simulink model "SLemba_CPG"  (R2024a)
settings: Solver=ode113  StartTime=0.0  StopTime=Sim.time  MaxStep=1e-3  RelTol=1e-5  AbsTol=1e-5
InitFcn:
  | parameters;
  | initBusObjects;
  | loadCPGParam;
undefined symbols (not defined in the file or in its folder): out
settings Model: Creator=heath  LastModifiedBy=Mechatronics
settings SolverCC: ZeroCrossControl=EnableAll
settings DebuggingCC: AlgebraicLoopMsg=none

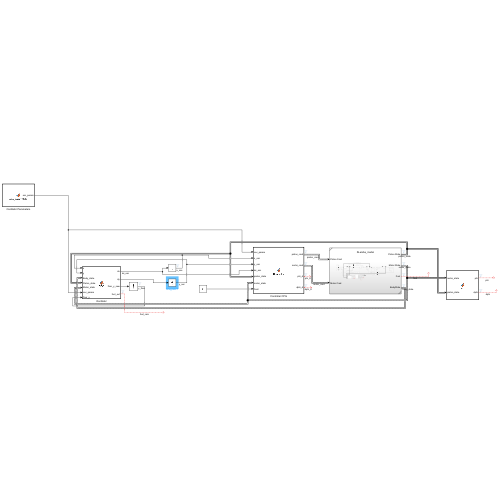
[thumbnail: Simulink's stored preview of the top-level diagram]
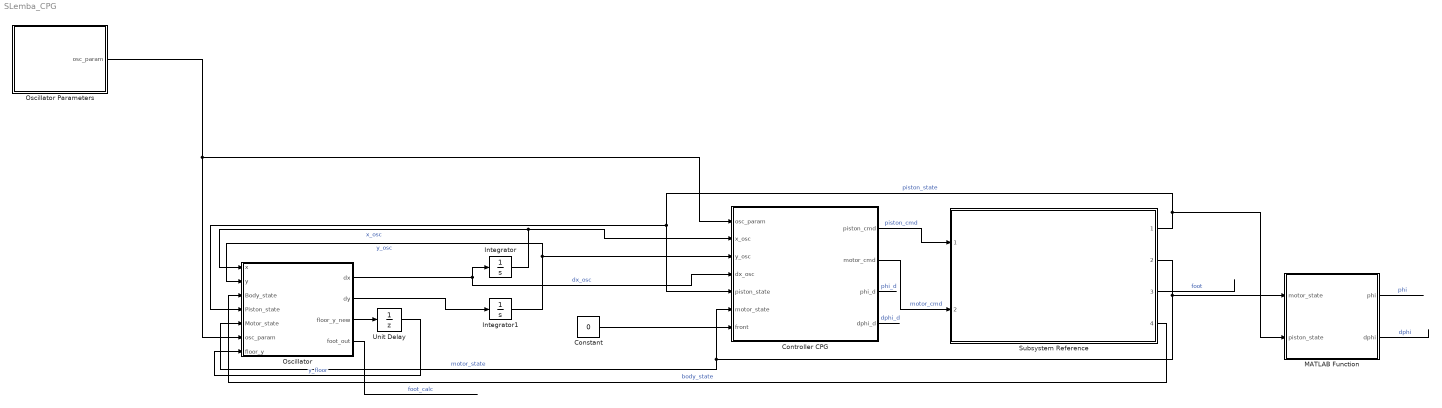
== system SLemba_CPG ==
  Constant : Constant  Value=0
  Controller CPG : MATLAB Function  TreatAsAtomicUnit=on
  Integrator : Integrator  InitialCondition=out.tstInit.CPG(1)
  Integrator1 : Integrator  InitialCondition=out.tstInit.CPG(2)
  MATLAB Function : MATLAB Function  TreatAsAtomicUnit=on
  Oscillator : MATLAB Function  TreatAsAtomicUnit=on
  Oscillator Parameters : MATLAB Function  TreatAsAtomicUnit=on
  Subsystem Reference : Subsystem  ReferencedSubsystem=SLemba_model
  Unit Delay : UnitDelay  SampleTime=-1  HasFrameUpgradeWarning=on
  wires:
  Integrator/1 -> Oscillator/1(x), Controller CPG/2(x_osc)  "x_osc"
  Integrator1/1 -> Oscillator/2(y), Controller CPG/3(y_osc)  "y_osc"
  Subsystem Reference/1 -> MATLAB Function/2(piston_state), Oscillator/4(Piston_state), Controller CPG/5(piston_state)  "piston_state"
  Subsystem Reference/2 -> MATLAB Function/1(motor_state), Oscillator/5(Motor_state), Controller CPG/6(motor_state)  "motor_state"
  Constant/1 -> Controller CPG/7(front)
  Controller CPG/1(piston_cmd) -> Subsystem Reference/1  "piston_cmd"
  Controller CPG/2(motor_cmd) -> Subsystem Reference/2  "motor_cmd"
  Subsystem Reference/4 -> Oscillator/3(Body_state)  "body_state"
  Subsystem Reference/3 -> ?  "foot"
  Controller CPG/3(phi_d) -> ?  "phi_d"
  Controller CPG/4(dphi_d) -> ?  "dphi_d"
  MATLAB Function/1(phi) -> ?  "phi"
  MATLAB Function/2(dphi) -> ?  "dphi"
  Oscillator/1(dx) -> Integrator/1, Controller CPG/4(dx_osc)  "dx_osc"
  Oscillator/2(dy) -> Integrator1/1
  Oscillator/3(floor_y_new) -> Unit Delay/1
  Unit Delay/1 -> Oscillator/7(floor_y)  "y_floor"
  Oscillator/4(foot_out) -> ?  "foot_calc"
  Oscillator Parameters/1(osc_param) -> Oscillator/6(osc_param), Controller CPG/1(osc_param)

== matlab function SLemba_CPG/Controller CPG ==
  data: osc_param input; x_osc input; piston_cmd output Bus: PistonCmd; y_osc input; dx_osc input; piston_state input PistonState; motor_state input MotorState; front input; motor_cmd output Bus: MotorCmd; phi_d output; dphi_d output
function [piston_cmd,motor_cmd,phi_d,dphi_d] = Controller(osc_param, x_osc,y_osc,dx_osc, piston_state,motor_state,front)

kx = osc_param(3);

l = piston_state.p;
dl = piston_state.v;
th = motor_state.q;

if (front)
    direction = -1;
else
    direction = 1;
end

% set command
phi_d = direction*x_osc*kx + pi/2;
dphi_d = direction*dx_osc*kx;
if (y_osc>0) 
    if(x_osc>0)
        ue = 0; ur = 1;
    else
            ue = 1; ur = 1;
    end
else
    ue = 1; ur = 0;
end

kp = 250;
kd = 10;

% % Testing
% % ----------
% ue = 0; ur = 0;
% phi_d = pi/2; dphi_d = 0;
% kp = 250;kd = 5;
% % ---------

piston_cmd.ue = ue;
piston_cmd.ur = ur;

motor_cmd.q = th_calc(phi_d,l);
motor_cmd.w = dth_calc(phi_calc(th,l),l,dphi_d,dl);
motor_cmd.Kp = kp;
motor_cmd.Kd = kd;
motor_cmd.tff = 0;

== matlab function SLemba_CPG/Oscillator ==
  data: x input size=1; dx output size=1; y input; Body_state input; Piston_state input; Motor_state input; osc_param input; dy output; floor_y_new output; floor_y input; foot_out output
function [dx,dy,floor_y_new,foot_out] = CPG(x,y,Body_state,Piston_state, Motor_state, osc_param,floor_y)%,dy_lift, fit)%dq_osc = CPG(input_osc)%
% x = input_osc.x_osc; y = input_osc.y_osc; osc_param = input_osc.osc_param;
% Body_state = input_osc.Body_state; Piston_state = input_osc.Piston_state; Motor_state = input_osc.Motor_state;

x_body = Body_state.x; y_body = Body_state.y;
dx_body = Body_state.dx; dy_body = Body_state.dy;
th = Motor_state.q; dth = Motor_state.w;
l = Piston_state.p; dl = Piston_state.v;

thk = thk_calc(th,l); tha = tha_calc(th,l);
dthk = dthk_calc(th,l,dth,dl); dtha = dtha_calc(th,l,dth,dl);

foot = foot_Func(x_body,y_body,th,l,thk,tha,dx_body,dy_body,dth,dl,dthk,dtha);

y_foot = foot(2);
dy_foot = foot(4);

% % update floor height based on piston impact
% piston_tol = -2e2;
% if (Piston_state.a < piston_tol)
%     floor_y = y_foot;
% end

y_foot = y_foot - floor_y;

foot(2) = y_foot;
foot_out = foot;

floor_y_new = floor_y;

tst = osc_param(1);
tsw = osc_param(2);

% constants
mu = 1;
F_1 = 50;
gamma = 10;
b = 100;


% if(dy_lift>0)
%     coeff = fit.coeff;
% 
%     tsw_new = coeff(1) + coeff(2)*tst + coeff(3)*dy_lift + coeff(4)*tst^2 + coeff(5)*tst*dy_lift + coeff(6)*dy_lift^2;
%     if (tsw_new>tst)
%         tsw = tsw_new;
%     end
% end


T = tst + tsw;
d = tsw/T;
% 
% % 3 frequencies with quadrant crossover
% omega_1 = pi/(T*d);
% omega_2 = omega_1;
% omega_3 = pi/(T - T*d);

k = 1; % 2 for extension at half way
e = 0;%0.4;

% 3 frequencies with quadrant crossover
omega_1 = (pi*k - 2*d*e + 2*d*e*k + pi)/(2*T*d*k);
omega_2 = k*omega_1;
omega_3 = (pi*k - 2*d*e + 2*d*e*k + pi)/(T - T*d + T*k - T*d*k);

% polar coordinates
r = sqrt(x^2 + y^2);
th = atan2(y,x);
% th = atan(y/x);
% if (x <= 0)
%     th = pi + atan(y/x);
% end

% 3 frequencies with quadrant cross over
k1 = omega_1/((exp(-b*(x))+1)*(exp(-b*y)+1));
k2 = omega_2/((exp(b*(x))+1)*(exp(-b*y)+1));
k3 = omega_3/(exp(b*y)+1);
omega = k1 + k2 + k3;

f = @(v) 1 + 0.5*cos(v)*tanh(sin(2*v));
f_dash = @(v) cos(v)*cos(2*v)*(sech(sin(2*v)))^2-0.5*sin(v)*tanh(sin(2*v));

% oscillation
dth = omega;
dr = mu*omega*f_dash(th) + gamma*(mu*f(th)-r);

% change in x
dx = dr*cos(th) - r*sin(th)*dth;

if (y_foot <= 0 && y > 0 && x < 0) % fast transition case 1
    u = -F_1;
elseif(y_foot > 0 && y < 0 && x > 0) % fast transition case 3
    u = F_1;
elseif (y < 0 && dy_foot < 0 && y_foot > 0) % slow transition case 2
    u = - omega*x;
else
    u = 0;
end

dy = dr*sin(th) + r*cos(th)*dth + u;

dq_osc.dx = dx;
dq_osc.dy = dy;
end

== matlab function SLemba_CPG/Oscillator Parameters ==
  data: osc_param output; CPG parameter
function osc_param = osc_paramCalc(CPG)

% persistent osc_paramVal
% 
% if isempty(osc_paramVal)
%     out = load("PSO_runs/sol.mat");
%     out = out.out;
%     tst = out.simParams.tst;
%     kx = out.simParams.kx;
% 
%     tsw = out.out.BestSol.Position(4);
% 
%     osc_paramVal = [tst,tsw,kx];
% end

tst = CPG.tst;
kx = CPG.kx;
tsw = CPG.tsw;

osc_param = [tst,tsw,kx];

== matlab function SLemba_CPG/MATLAB Function ==
  data: motor_state input; phi output; piston_state input; dphi output
function [phi,dphi] = fcn(motor_state,piston_state)

phi = phi_calc(motor_state.q,piston_state.p);
dphi = dphi_calc(motor_state.q,piston_state.p,motor_state.w,piston_state.v);
